simulink model "jpeg"  (R2022b)
settings: Solver=FixedStepDiscrete  StartTime=0.0  StopTime=0.01  RelTol=1e-3
undefined symbols (not defined in the file): gray, HDTV, M, N, Rec, sz
libraries: vipmisc x9, visionconversions x7, visiontransforms x6, visionsources x1
settings Model: Creator=15pra  LastModifiedBy=15pra
settings SolverCC: AlgebraicLoopSolver=TrustRegion  AutoInsertRateTranBlk=on
settings DataIOCC: LimitDataPoints=on  SaveOutput=off  SignalLogging=off  SaveTime=off
settings OptimizationCC: LifeSpan=inf  SimCompilerOptimization=on
settings DebuggingCC: AlgebraicLoopMsg=error  SingleTaskRateTransMsg=error  UnconnectedInputMsg=warning  UnconnectedOutputMsg=warning  UnconnectedLineMsg=warning  AllowSymbolicDim=off  SFUnexpectedBacktrackingDiag=warning  SFNoUnconditionalDefaultTransitionDiag=warning  SFExecutionAtInitializationDiag=none  SFMachineParentedDataDiag=warning  ArithmeticOperatorsInVariantConditions=warning
settings ModelReferenceCC: EnableRefExpFcnMdlSchedulingChecks=on
settings SFSimCC: SimUseLocalCustomCode=off  CustomCodeUndefinedFunction=UseInterfaceOnly
settings RTWCC: RTWUseLocalCustomCode=off
settings CodeAppCC: StateflowObjectComments=on
settings GRTTargetCC: TargetLangStandard=C89/C90 (ANSI)
settings ConfigComp: CovMetricSettings=dw  CovSaveCumulativeToWorkspaceVar=on  CovSaveSingleToWorkspaceVar=on  CovExternalEMLEnable=off  CovSFcnEnable=off

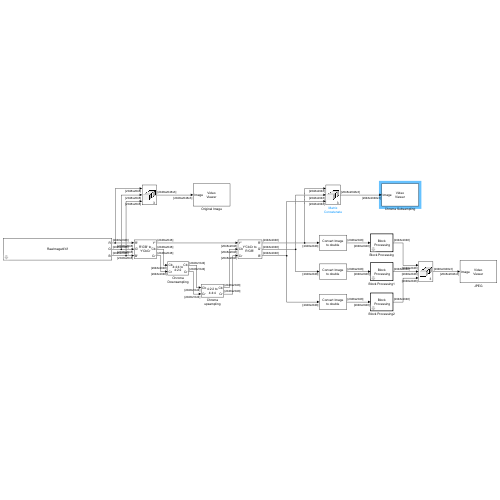
[thumbnail: Simulink's stored preview of the top-level diagram]
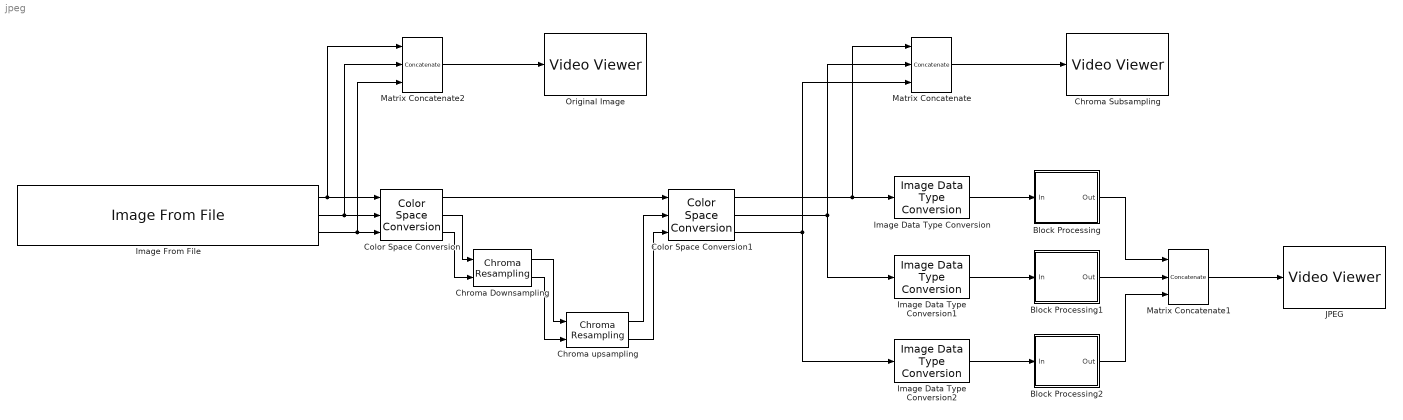
== system jpeg ==
  Block Processing : Subsystem  TreatAsAtomicUnit=on  mask(Block Processing){NumI=1, ParamPort=off, NumO=1, Blocksize={[8 8]}, Overlapsize={[0 0]}, Traverse=Row-wise}
      mask prompts: NumI "vision:masks:NumberOfInputs"; ParamPort "vision:masks:AddPortToSupplySubsystemParam"; NumO "vision:masks:NumberOfOutputs"; Blocksize "vision:masks:BlockSize"; Overlapsize "vision:masks:OverlapSize"; Traverse "vision:masks:TraverseOrder"
      mask help: vision:masks:BlockProcessingDescription
      mask init:
      | errmsg = vipblkblockproc(gcbh, NumI, NumO, Blocksize, Overlapsize, Traverse, ParamPort);
      | error(errmsg);
      settings: CopyFcn=set_param(gcb,'LinkStatus','none');
      mask Help: eval('helpview(fullfile(docroot,''toolbox'',''vision'',''vision.map''),''visionblockprocessing'')');
      mask TypeOptions Traverse: vision:masks:Rowwise | vision:masks:Columnwise
      mask DialogControl NumI Prompt: Number of inputs:
      mask DialogControl ParamPort Prompt: Add port to supply subsystem parameters
      mask DialogControl NumO Prompt: Number of outputs:
      mask DialogControl Blocksize Prompt: Block size:
      mask DialogControl Overlapsize Prompt: Overlap size:
      mask DialogControl Traverse Prompt: Traverse order:
      mask DialogControl subsystemGrpBox Prompt: vision:masks:Subsystem
      mask DialogControl subsystemText Prompt: vision:masks:ClickTheOpenSubsystemButton
      mask DialogControl openSubsystem Prompt: vision:masks:OpenSubsystem
      mask DialogControl openSubsystem Callback: Opensubsystem(gcbh)
      mask Display:
      | disp('Block\n Processing');
      | 
      | if ((NumI == 1) && ParamPort)
      |     port_label('input', 1, 'I');
      | end
      | 
      | if (NumI > 1)
      |     for (i = 1:NumI)
      |         port_label('input', i, ['I' int2str(i)]);
      |     end
      | end
      | 
      | if (ParamPort)
      |     port_label('input', NumI+1, 'P');
      | end
  Block Processing1 : Subsystem  TreatAsAtomicUnit=on  mask(Block Processing){NumI=1, ParamPort=off, NumO=1, Blocksize={[8 8]}, Overlapsize={[0 0]}, Traverse=Row-wise}
      mask prompts: NumI "vision:masks:NumberOfInputs"; ParamPort "vision:masks:AddPortToSupplySubsystemParam"; NumO "vision:masks:NumberOfOutputs"; Blocksize "vision:masks:BlockSize"; Overlapsize "vision:masks:OverlapSize"; Traverse "vision:masks:TraverseOrder"
      mask help: vision:masks:BlockProcessingDescription
      mask init:
      | errmsg = vipblkblockproc(gcbh, NumI, NumO, Blocksize, Overlapsize, Traverse, ParamPort);
      | error(errmsg);
      settings: CopyFcn=set_param(gcb,'LinkStatus','none');
      mask Help: eval('helpview(fullfile(docroot,''toolbox'',''vision'',''vision.map''),''visionblockprocessing'')');
      mask TypeOptions Traverse: vision:masks:Rowwise | vision:masks:Columnwise
      mask DialogControl NumI Prompt: Number of inputs:
      mask DialogControl ParamPort Prompt: Add port to supply subsystem parameters
      mask DialogControl NumO Prompt: Number of outputs:
      mask DialogControl Blocksize Prompt: Block size:
      mask DialogControl Overlapsize Prompt: Overlap size:
      mask DialogControl Traverse Prompt: Traverse order:
      mask DialogControl subsystemGrpBox Prompt: vision:masks:Subsystem
      mask DialogControl subsystemText Prompt: vision:masks:ClickTheOpenSubsystemButton
      mask DialogControl openSubsystem Prompt: vision:masks:OpenSubsystem
      mask DialogControl openSubsystem Callback: Opensubsystem(gcbh)
      mask Display:
      | disp('Block\n Processing');
      | 
      | if ((NumI == 1) && ParamPort)
      |     port_label('input', 1, 'I');
      | end
      | 
      | if (NumI > 1)
      |     for (i = 1:NumI)
      |         port_label('input', i, ['I' int2str(i)]);
      |     end
      | end
      | 
      | if (ParamPort)
      |     port_label('input', NumI+1, 'P');
      | end
  Block Processing2 : Subsystem  TreatAsAtomicUnit=on  mask(Block Processing){NumI=1, ParamPort=off, NumO=1, Blocksize={[8 8]}, Overlapsize={[0 0]}, Traverse=Row-wise}
      mask prompts: NumI "vision:masks:NumberOfInputs"; ParamPort "vision:masks:AddPortToSupplySubsystemParam"; NumO "vision:masks:NumberOfOutputs"; Blocksize "vision:masks:BlockSize"; Overlapsize "vision:masks:OverlapSize"; Traverse "vision:masks:TraverseOrder"
      mask help: vision:masks:BlockProcessingDescription
      mask init:
      | errmsg = vipblkblockproc(gcbh, NumI, NumO, Blocksize, Overlapsize, Traverse, ParamPort);
      | error(errmsg);
      settings: CopyFcn=set_param(gcb,'LinkStatus','none');
      mask Help: eval('helpview(fullfile(docroot,''toolbox'',''vision'',''vision.map''),''visionblockprocessing'')');
      mask TypeOptions Traverse: vision:masks:Rowwise | vision:masks:Columnwise
      mask DialogControl NumI Prompt: Number of inputs:
      mask DialogControl ParamPort Prompt: Add port to supply subsystem parameters
      mask DialogControl NumO Prompt: Number of outputs:
      mask DialogControl Blocksize Prompt: Block size:
      mask DialogControl Overlapsize Prompt: Overlap size:
      mask DialogControl Traverse Prompt: Traverse order:
      mask DialogControl subsystemGrpBox Prompt: vision:masks:Subsystem
      mask DialogControl subsystemText Prompt: vision:masks:ClickTheOpenSubsystemButton
      mask DialogControl openSubsystem Prompt: vision:masks:OpenSubsystem
      mask DialogControl openSubsystem Callback: Opensubsystem(gcbh)
      mask Display:
      | disp('Block\n Processing');
      | 
      | if ((NumI == 1) && ParamPort)
      |     port_label('input', 1, 'I');
      | end
      | 
      | if (NumI > 1)
      |     for (i = 1:NumI)
      |         port_label('input', i, ['I' int2str(i)]);
      |     end
      | end
      | 
      | if (ParamPort)
      |     port_label('input', NumI+1, 'P');
      | end
  Chroma Downsampling : visionconversions/Chroma Resampling  resampling=4:4:4 to 4:2:2  interpolation=linear  antialiasing=Default  hcoeff=[0.2 0.6 0.2]  vcoeff=[0.5 0.5]  isInputTransposed=off
  Chroma upsampling : visionconversions/Chroma Resampling  resampling=4:2:2 to 4:4:4  interpolation=linear  antialiasing=Default  hcoeff=[0.2 0.6 0.2]  vcoeff=[0.5 0.5]  isInputTransposed=off
  Chroma Subsampling : VideoViewer  colormapValue=gray(256)  FigPos=[505 664.4 430.4 441.6]
  Color Space Conversion : visionconversions/Color Space  Conversion  conversion=Obsolete  conversionActive=R'G'B' to Y'CbCr  wp_str=D65  rec=Rec. 709 (HDTV)  sys=1125/60/2:1  imagePorts=Separate color signals
  Color Space Conversion1 : visionconversions/Color Space  Conversion  conversion=Obsolete  conversionActive=Y'CbCr to R'G'B'  wp_str=D65  rec=Rec. 709 (HDTV)  sys=1125/60/2:1  imagePorts=Separate color signals
  Image Data Type Conversion : visionconversions/Image Data Type Conversion  outDT=double  isSigned=on  wordLen=16  numFracBits=0
  Image Data Type Conversion1 : visionconversions/Image Data Type Conversion  outDT=double  isSigned=on  wordLen=16  numFracBits=0
  Image Data Type Conversion2 : visionconversions/Image Data Type Conversion  outDT=double  isSigned=on  wordLen=16  numFracBits=0
  Image From File : visionsources/Image From File  Tag=vipblks_nd  FileName=D:\Study Material\Sem 6\Digital Signal Proscessing\Rawimagetif.tif  Ts=inf  imagePorts=Separate color signals  OutPortLabels=R|G|B  ImageDataType=uint8  sdImageDataType=uint(8)  Signed=on  WordLength=16  FractionLengthMode=User-defined  FractionLength=15
  JPEG : VideoViewer  colormapValue=gray(256)  FigPos=[941.8 662.8 431.2 440.8]
  Matrix Concatenate : Concatenate  NumInputs=3  Mode=Multidimensional array  ConcatenateDimension=3
  Matrix Concatenate1 : Concatenate  NumInputs=3  Mode=Multidimensional array  ConcatenateDimension=3
  Matrix Concatenate2 : Concatenate  NumInputs=3  Mode=Multidimensional array  ConcatenateDimension=3
  Original Image : VideoViewer  colormapValue=gray(256)  FigPos=[69 662.8 430.4 441.6]
  wires:
  Color Space Conversion/2 -> Chroma Downsampling/1
  Color Space Conversion/3 -> Chroma Downsampling/2
  Color Space Conversion/1 -> Color Space Conversion1/1
  Chroma Downsampling/1 -> Chroma upsampling/1
  Chroma Downsampling/2 -> Chroma upsampling/2
  Chroma upsampling/1 -> Color Space Conversion1/2
  Chroma upsampling/2 -> Color Space Conversion1/3
  Color Space Conversion1/1 -> Matrix Concatenate/1, Image Data Type Conversion/1
  Color Space Conversion1/2 -> Image Data Type Conversion1/1, Matrix Concatenate/2
  Color Space Conversion1/3 -> Image Data Type Conversion2/1, Matrix Concatenate/3
  Image From File/1 -> Matrix Concatenate2/1, Color Space Conversion/1
  Image From File/2 -> Matrix Concatenate2/2, Color Space Conversion/2
  Matrix Concatenate/1 -> Chroma Subsampling/1
  Image From File/3 -> Matrix Concatenate2/3, Color Space Conversion/3
  Image Data Type Conversion/1 -> Block Processing/1(In)
  Image Data Type Conversion1/1 -> Block Processing1/1(In)
  Image Data Type Conversion2/1 -> Block Processing2/1(In)
  Matrix Concatenate1/1 -> JPEG/1
  Block Processing/1(Out) -> Matrix Concatenate1/1
  Block Processing1/1(Out) -> Matrix Concatenate1/2
  Block Processing2/1(Out) -> Matrix Concatenate1/3
  Matrix Concatenate2/1 -> Original Image/1

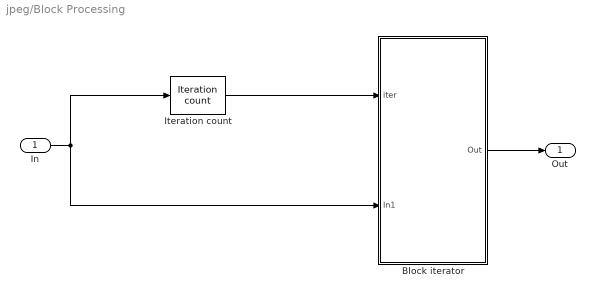
== system jpeg/Block Processing ==
  In : Inport
  Block iterator : Subsystem
      settings: CopyFcn=set_param(gcb,'ReferenceBlock','');
  Iteration count : vipmisc/Iteration count  NumI=NumI  blksize=Blocksize  ovlpsize=Overlapsize
  Out : Outport  VectorParamsAs1DForOutWhenUnconnected=off
  wires:
  Iteration count/1 -> Block iterator/1(iter)
  In/1 -> Iteration count/1, Block iterator/2(In1)
  Block iterator/1(Out) -> Out/1

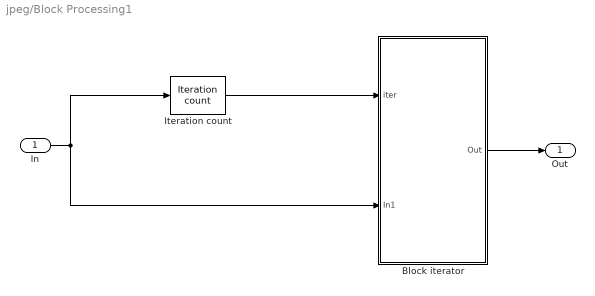
== system jpeg/Block Processing1 ==
  In : Inport
  Block iterator : Subsystem
      settings: CopyFcn=set_param(gcb,'ReferenceBlock','');
  Iteration count : vipmisc/Iteration count  NumI=NumI  blksize=Blocksize  ovlpsize=Overlapsize
  Out : Outport  VectorParamsAs1DForOutWhenUnconnected=off
  wires:
  Iteration count/1 -> Block iterator/1(iter)
  In/1 -> Iteration count/1, Block iterator/2(In1)
  Block iterator/1(Out) -> Out/1

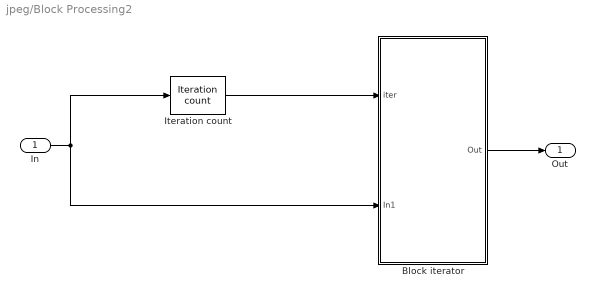
== system jpeg/Block Processing2 ==
  In : Inport
  Block iterator : Subsystem
      settings: CopyFcn=set_param(gcb,'ReferenceBlock','');
  Iteration count : vipmisc/Iteration count  NumI=NumI  blksize=Blocksize  ovlpsize=Overlapsize
  Out : Outport  VectorParamsAs1DForOutWhenUnconnected=off
  wires:
  Iteration count/1 -> Block iterator/1(iter)
  In/1 -> Iteration count/1, Block iterator/2(In1)
  Block iterator/1(Out) -> Out/1

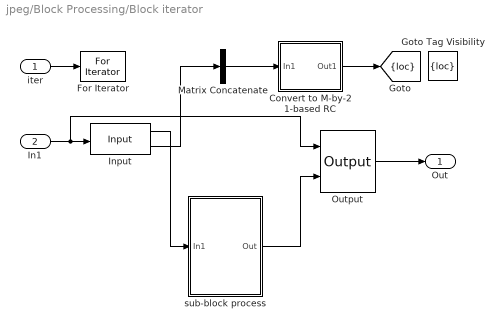
== system jpeg/Block Processing/Block iterator ==
  iter : Inport
  In1 : Inport  Port=2
  Convert to M-by-2 1-based RC : Subsystem
  For Iterator : ForIterator  IterationSource=external  IterationLimit=(sz(1)/M)*(sz(2)/N)  ShowIterationPort=off  IndexMode=Zero-based  IterationVariableDataType=double
  Goto Tag Visibility : GotoTagVisibility  GotoTag=loc
  Input : vipmisc/Input  Blocksize=Blocksize{1}  Overlapsize=Overlapsize{1}  tverse=Row-wise
  Matrix Concatenate : Concatenate  NumInputs=1  Mode=Multidimensional array  ConcatenateDimension=2
  Output : vipmisc/Output  Blocksize=Blocksize{1}  Overlapsize=Overlapsize{1}  tverse=Row-wise
  sub-block process : Subsystem
  Out : Outport  VectorParamsAs1DForOutWhenUnconnected=off
  tag scope: loc=scoped
  wires:
  Convert to M-by-2 1-based RC/1(Out1) -> [loc]
  Matrix Concatenate/1 -> Convert to M-by-2 1-based RC/1(In1)
  Input/2 -> Matrix Concatenate/1
  Input/1 -> sub-block process/1(In1)
  iter/1 -> For Iterator/1
  In1/1 -> Input/1, Output/1
  Output/1 -> Out/1
  sub-block process/1(Out) -> Output/2

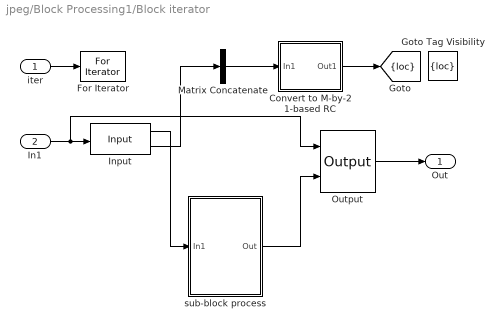
== system jpeg/Block Processing1/Block iterator ==
  iter : Inport
  In1 : Inport  Port=2
  Convert to M-by-2 1-based RC : Subsystem
  For Iterator : ForIterator  IterationSource=external  IterationLimit=(sz(1)/M)*(sz(2)/N)  ShowIterationPort=off  IndexMode=Zero-based  IterationVariableDataType=double
  Goto Tag Visibility : GotoTagVisibility  GotoTag=loc
  Input : vipmisc/Input  Blocksize=Blocksize{1}  Overlapsize=Overlapsize{1}  tverse=Row-wise
  Matrix Concatenate : Concatenate  NumInputs=1  Mode=Multidimensional array  ConcatenateDimension=2
  Output : vipmisc/Output  Blocksize=Blocksize{1}  Overlapsize=Overlapsize{1}  tverse=Row-wise
  sub-block process : Subsystem
  Out : Outport  VectorParamsAs1DForOutWhenUnconnected=off
  tag scope: loc=scoped
  wires:
  Convert to M-by-2 1-based RC/1(Out1) -> [loc]
  Matrix Concatenate/1 -> Convert to M-by-2 1-based RC/1(In1)
  Input/2 -> Matrix Concatenate/1
  Input/1 -> sub-block process/1(In1)
  iter/1 -> For Iterator/1
  In1/1 -> Input/1, Output/1
  Output/1 -> Out/1
  sub-block process/1(Out) -> Output/2

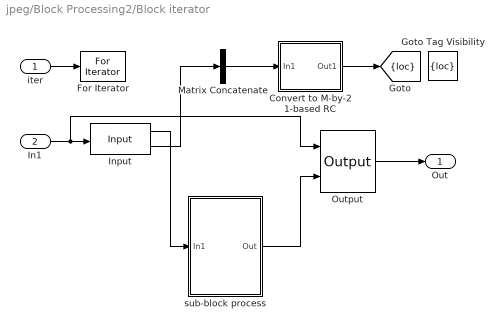
== system jpeg/Block Processing2/Block iterator ==
  iter : Inport
  In1 : Inport  Port=2
  Convert to M-by-2 1-based RC : Subsystem
  For Iterator : ForIterator  IterationSource=external  IterationLimit=(sz(1)/M)*(sz(2)/N)  ShowIterationPort=off  IndexMode=Zero-based  IterationVariableDataType=double
  Goto Tag Visibility : GotoTagVisibility  GotoTag=loc
  Input : vipmisc/Input  Blocksize=Blocksize{1}  Overlapsize=Overlapsize{1}  tverse=Row-wise
  Matrix Concatenate : Concatenate  NumInputs=1  Mode=Multidimensional array  ConcatenateDimension=2
  Output : vipmisc/Output  Blocksize=Blocksize{1}  Overlapsize=Overlapsize{1}  tverse=Row-wise
  sub-block process : Subsystem
  Out : Outport  VectorParamsAs1DForOutWhenUnconnected=off
  tag scope: loc=scoped
  wires:
  Convert to M-by-2 1-based RC/1(Out1) -> [loc]
  Matrix Concatenate/1 -> Convert to M-by-2 1-based RC/1(In1)
  Input/2 -> Matrix Concatenate/1
  Input/1 -> sub-block process/1(In1)
  iter/1 -> For Iterator/1
  In1/1 -> Input/1, Output/1
  Output/1 -> Out/1
  sub-block process/1(Out) -> Output/2

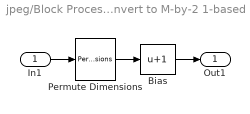
== system jpeg/Block Processing/Block iterator/Convert to M-by-2 1-based RC ==
  In1 : Inport
  Bias : Bias  Bias=1  SaturateOnIntegerOverflow=off
  Permute Dimensions : PermuteDimensions
  Out1 : Outport  VectorParamsAs1DForOutWhenUnconnected=off
  wires:
  In1/1 -> Permute Dimensions/1
  Bias/1 -> Out1/1
  Permute Dimensions/1 -> Bias/1

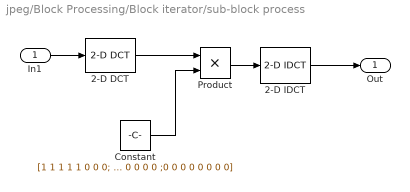
== system jpeg/Block Processing/Block iterator/sub-block process ==
  In1 : Inport
  2-D DCT : visiontransforms/2-D DCT  CompMethod=Table lookup  Dimension=0  TableOpt=Speed  BitRevOrder=off  SkipNorm=off  firstCoeffLastDataTypeStr=Inherit: Same word length as input  roundingMode=Floor  overflowMode=off  firstCoeffDataTypeStr=Inherit: Same word length as input  outputMin=[]  outputMax=[]
  2-D IDCT : visiontransforms/2-D IDCT  CompMethod=Table lookup  Dimension=0  TableOpt=Speed  BitRevOrder=off  SkipNorm=off  firstCoeffLastDataTypeStr=Inherit: Same word length as input  roundingMode=Floor  overflowMode=off  firstCoeffDataTypeStr=Inherit: Same word length as input  outputMin=[]  outputMax=[]
  Constant : Constant  Value=[1 1 1 1 1 0 0 0; 1 1 1 1 0 0 0 0; 1 1 1 0 0 0 0 0; 1 1 0 0 0 0 0 0; 1 0 0 0 0 0 0 0; 0 0 0 0 0 0 0 0; 0 0 0 0 0 0 0 0 ;0 0 0 0 0 0 0 0]  VectorParams1D=off
  Product : Product
  Out : Outport  VectorParamsAs1DForOutWhenUnconnected=off
  wires:
  2-D DCT/1 -> Product/1
  Constant/1 -> Product/2
  Product/1 -> 2-D IDCT/1
  2-D IDCT/1 -> Out/1
  In1/1 -> 2-D DCT/1

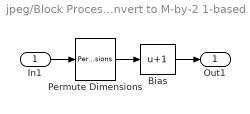
== system jpeg/Block Processing1/Block iterator/Convert to M-by-2 1-based RC ==
  In1 : Inport
  Bias : Bias  Bias=1  SaturateOnIntegerOverflow=off
  Permute Dimensions : PermuteDimensions
  Out1 : Outport  VectorParamsAs1DForOutWhenUnconnected=off
  wires:
  In1/1 -> Permute Dimensions/1
  Bias/1 -> Out1/1
  Permute Dimensions/1 -> Bias/1

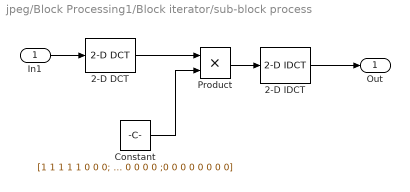
== system jpeg/Block Processing1/Block iterator/sub-block process ==
  In1 : Inport
  2-D DCT : visiontransforms/2-D DCT  CompMethod=Table lookup  Dimension=0  TableOpt=Speed  BitRevOrder=off  SkipNorm=off  firstCoeffLastDataTypeStr=Inherit: Same word length as input  roundingMode=Floor  overflowMode=off  firstCoeffDataTypeStr=Inherit: Same word length as input  outputMin=[]  outputMax=[]
  2-D IDCT : visiontransforms/2-D IDCT  CompMethod=Table lookup  Dimension=0  TableOpt=Speed  BitRevOrder=off  SkipNorm=off  firstCoeffLastDataTypeStr=Inherit: Same word length as input  roundingMode=Floor  overflowMode=off  firstCoeffDataTypeStr=Inherit: Same word length as input  outputMin=[]  outputMax=[]
  Constant : Constant  Value=[1 1 1 1 1 0 0 0; 1 1 1 1 0 0 0 0; 1 1 1 0 0 0 0 0; 1 1 0 0 0 0 0 0; 1 0 0 0 0 0 0 0; 0 0 0 0 0 0 0 0; 0 0 0 0 0 0 0 0 ;0 0 0 0 0 0 0 0]  VectorParams1D=off
  Product : Product
  Out : Outport  VectorParamsAs1DForOutWhenUnconnected=off
  wires:
  2-D DCT/1 -> Product/1
  Constant/1 -> Product/2
  Product/1 -> 2-D IDCT/1
  2-D IDCT/1 -> Out/1
  In1/1 -> 2-D DCT/1

== system jpeg/Block Processing2/Block iterator/Convert to M-by-2 1-based RC ==
  In1 : Inport
  Bias : Bias  Bias=1  SaturateOnIntegerOverflow=off
  Permute Dimensions : PermuteDimensions
  Out1 : Outport  VectorParamsAs1DForOutWhenUnconnected=off
  wires:
  In1/1 -> Permute Dimensions/1
  Bias/1 -> Out1/1
  Permute Dimensions/1 -> Bias/1

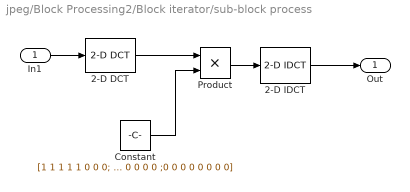
== system jpeg/Block Processing2/Block iterator/sub-block process ==
  In1 : Inport
  2-D DCT : visiontransforms/2-D DCT  CompMethod=Table lookup  Dimension=0  TableOpt=Speed  BitRevOrder=off  SkipNorm=off  firstCoeffLastDataTypeStr=Inherit: Same word length as input  roundingMode=Floor  overflowMode=off  firstCoeffDataTypeStr=Inherit: Same word length as input  outputMin=[]  outputMax=[]
  2-D IDCT : visiontransforms/2-D IDCT  CompMethod=Table lookup  Dimension=0  TableOpt=Speed  BitRevOrder=off  SkipNorm=off  firstCoeffLastDataTypeStr=Inherit: Same word length as input  roundingMode=Floor  overflowMode=off  firstCoeffDataTypeStr=Inherit: Same word length as input  outputMin=[]  outputMax=[]
  Constant : Constant  Value=[1 1 1 1 1 0 0 0; 1 1 1 1 0 0 0 0; 1 1 1 0 0 0 0 0; 1 1 0 0 0 0 0 0; 1 0 0 0 0 0 0 0; 0 0 0 0 0 0 0 0; 0 0 0 0 0 0 0 0 ;0 0 0 0 0 0 0 0]  VectorParams1D=off
  Product : Product
  Out : Outport  VectorParamsAs1DForOutWhenUnconnected=off
  wires:
  2-D DCT/1 -> Product/1
  Constant/1 -> Product/2
  Product/1 -> 2-D IDCT/1
  2-D IDCT/1 -> Out/1
  In1/1 -> 2-D DCT/1
